simulink model "test_kinematic_model"  (R2019b)
settings: Solver=VariableStepAuto  StartTime=0.0  StopTime=10  RelTol=1e-3
libraries: simulink x1
settings Model: Creator=jiyo  LastModifiedBy=jiyo

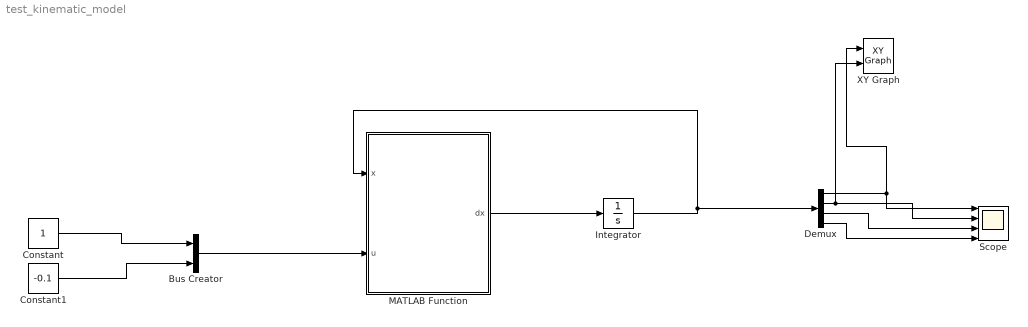
== system test_kinematic_model ==
  Bus Creator : BusCreator  Inputs=2
  Constant : Constant  OutDataTypeStr=double
  Constant1 : Constant  Value=-0.1  OutDataTypeStr=double
  Demux : Demux
  Integrator : Integrator  InitialCondition=[0.0 0.0 0.0 0.0]
  MATLAB Function : MATLAB Function  TreatAsAtomicUnit=on
  Scope : Scope  NumInputPorts=4
  XY Graph : simulink/Sinks/XY Graph  xmin=-30  xmax=30  ymin=-30  ymax=30  st=-1
  wires:
  MATLAB Function/1(dx) -> Integrator/1
  Integrator/1 -> Demux/1, MATLAB Function/1(x)
  Bus Creator/1 -> MATLAB Function/2(u)
  Constant/1 -> Bus Creator/1
  Constant1/1 -> Bus Creator/2
  Demux/1 -> Scope/1, XY Graph/1
  Demux/2 -> Scope/2, XY Graph/2
  Demux/3 -> Scope/3
  Demux/4 -> Scope/4

== matlab function test_kinematic_model/MATLAB Function ==
  data: x input; u input; dx output
function dx = fcn(x,u)
dx = vkinematicmodel_bicycle(x,u);
